simulink model "design_sim"  (R2023b)
settings: Solver=VariableStepAuto  StartTime=0.0  StopTime=1  MaxStep=1e-3  RelTol=1e-3
values from neighbouring files (symbols this model uses):
  b_int = round(b*(2^15))'    [design.m]
settings Model: Creator=fabiancastano  LastModifiedBy=fabiancastano

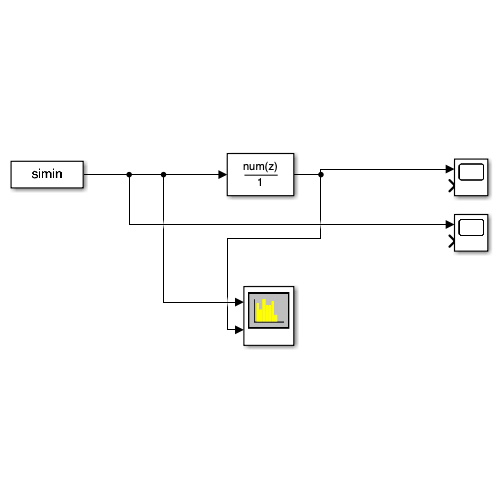
[thumbnail: Simulink's stored preview of the top-level diagram]
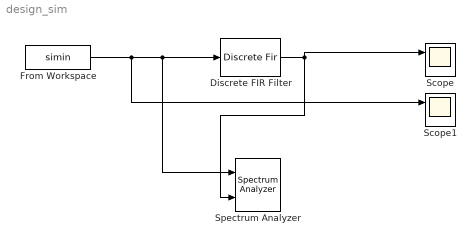
== system design_sim ==
  Discrete FIR Filter : DiscreteFir  Coefficients=b_int
  From Workspace : FromWorkspace  VariableName=simin  SampleTime=-1
  Scope : Scope  NumInputPorts=2
  Scope1 : Scope  NumInputPorts=2
  Spectrum Analyzer : SpectrumAnalyzer  NumInputPorts=2  WindowPosition=[320.000000,200.000000,800.000000,500.000000,]  ScopeFrameLocation=window  SampleRate=500  PlotAsTwoSidedSpectrum=off  Span=250  CenterFrequency=125  StartFrequency=0  StopFrequency=250  YLimits=[-184.8632191,50.52365506]  ColorLimits=[-233.20305566,50.86214921]
      settings: OpenAtSimulationStart=off
  wires:
  From Workspace/1 -> Scope1/1, Discrete FIR Filter/1, Spectrum Analyzer/1
  Discrete FIR Filter/1 -> Spectrum Analyzer/2, Scope/1
